simulink model "Wind_Turbine_test"  (R2023b)
settings: Solver=VariableStepAuto  StartTime=0.0  StopTime=1  RelTol=1e-3
model workspace (MAT data in the model file):
  Compensation_Ki = 30
  Compensation_Kp = 3
  DC_Ki = 400
  DC_Kp = 8
  F = 0.01
  Flux_min = 0.5
  Grid_Freq_PWM = 2700
  Grid_Ireg_Ki = 5
  Grid_Ireg_Kp = 0.83
  Grid_Ireg_lim = 1.1
  Grid_Modindex_Upper = 1.1
  Grid_conv_Imax = 0.8
  H = 0.685
  Idref_max = 0.9
  Iqref_Tc = 0.3
  Ki_Var = 0.05
  Ki_Vreg = 20
  Ksh = 1.1
  L_pu = 0.3
  Llr = 0.16
  Lls = 0.18
  Lm = 2.9
  P_mech = 1080000
  Pitch_Ki = 0
  Pitch_Kp = 150
  Pitch_Max = 27
  Pitch_Tc = 0.01
  Pitch_rate = 10
  Q_Filt = 50
  R_pu = 0.003
  Rotor_Freq_PWM = 1620
  Rotor_Ireg_Ki = 8
  Rotor_Ireg_Kp = 0.6
  Rotor_Ireg_lim = 0.1
  Rotor_Modindex_Upper = 2
  Rr = 0.016
  Rs = 0.023
  T_set = 0.0001
  Tp = 5e-05
  Ts = 5e-06
  Var_C_Filt = 720000
  Var_reg_max = 1.1
  Var_reg_min = 0.9
  WT_Coeff = [0.645 116 0.4 5 21 0.00912 0.08 0.035]
  WT_H = 4.32
  WT_IGBTRon = 5.931
  WT_Param = [91.204 10143]
  Wind_Freq_Filt = 10000
  Wind_Freq_nom = 60
  Wind_P_nom = 1200000
  Wind_Rotor_V_nom = 1950
  Wind_V_nom = 500
  Zeta_Filt = 0.707106781187
  init = [-0.2 0 0 0 0 0 0 0]
  p = 3
  torque0 = 0.83
  v_Ki = 0.1
  v_Kp = 3.6
  v_Max = 1.2
  v_Min = 0.7
  v_T = 5
  vreg_max = 1
  wind_VDC_nom = 1150
  wt0 = 1.2
undefined symbols (not defined in the file): D1, D11, Delta, DiscIntNeverNeededParam, P, Q
libraries: powerlib_extras x144, simulink_extras x24, spsThreePhaseVIMeasurementLib x13, spsThreePhaseTransformerTwoWindingsLib x11, spsSeriesRLCBranchLib x9, spsPWMGenerator2LevelLib x8, spsUniversalBridgeLib x8, spsThreePhaseSeriesRLCLoadLib x6, spsThreePhasePISectionLineLib x5, spsGroundLib x5, spsLoadFlowBusLib x4, spsAsynchronousMachinepuUnitsLib x4
(part 1 of 9)
settings Model: Creator=3.22  LastModifiedBy=3.22

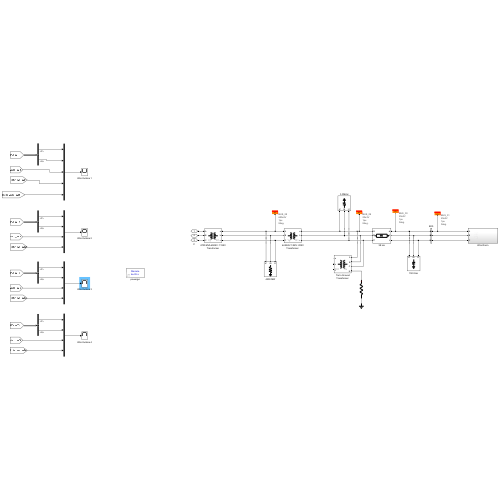
[thumbnail: Simulink's stored preview of the top-level diagram]
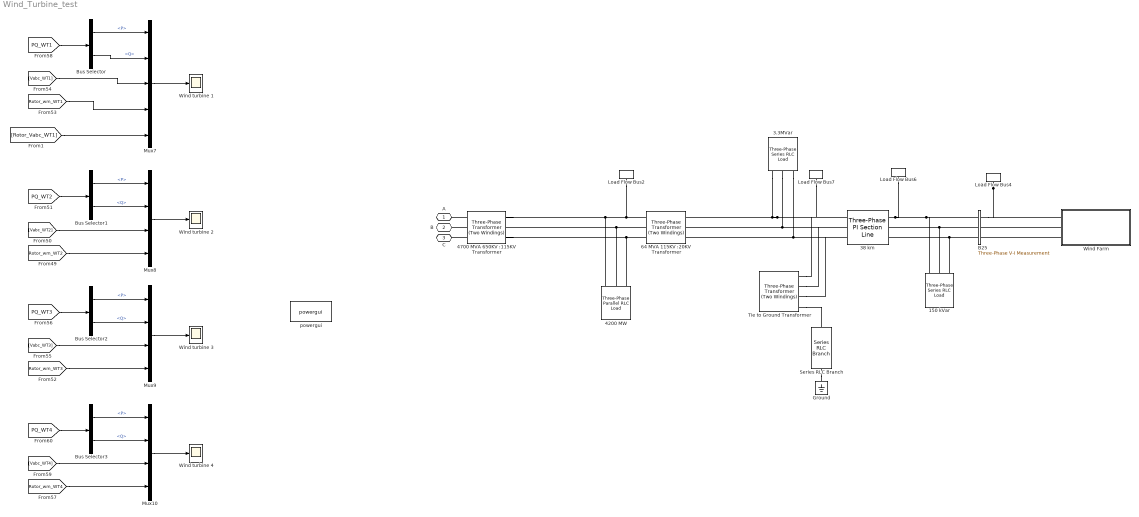
== system Wind_Turbine_test ==
  " 64 MVA 115KV :20KV Transformer " : spsThreePhaseTransformerTwoWindingsLib/Three-Phase Transformer (Two Windings)  Winding1Connection=Yg  Winding2Connection=Delta (D1)  CoreType=Three single-phase transformers  SetSaturation=off  Hysteresis=off  DataFile='hysteresis'  SetInitialFlux=off  Measurements=None  UNITS=pu  NominalPower=[ 64e6 , 60 ]  Winding1=[ 115e3 , 0.002 , 0.08 ]  Winding2=[ 20e3 , 0.002 , 0.08 ]  Rm=500  Lm=500  L0=0.5  Saturation=[ 0,0 ; 0.0024,1.2 ; 1.0,1.52 ]  InitialFluxes=[ 0.8 , -0.8 , 0.7 ]  BreakLoop=off  DiscreteSolver=Trapezoidal iterative  DataType=off  TransfoNumber=1
  " Tie to Ground Transformer " : spsThreePhaseTransformerTwoWindingsLib/Three-Phase Transformer (Two Windings)  Winding1Connection=Yn  Winding2Connection=Delta (D11)  CoreType=Three single-phase transformers  SetSaturation=off  Hysteresis=off  DataFile='hysteresis'  SetInitialFlux=off  Measurements=None  UNITS=pu  NominalPower=[ 5600e6 , 60 ]  Winding1=[ 13.8e3 , 0.002 , 0.08 ]  Winding2=[ 735e3 , 0.002 , 0.08 ]  Rm=500  Lm=500  L0=0.5  Saturation=[ 0,0 ; 0.0024,1.2 ; 1.0,1.52 ]  InitialFluxes=[ 0.8 , -0.8 , 0.7 ]  BreakLoop=off  DiscreteSolver=Trapezoidal iterative  DataType=off  TransfoNumber=1
  150 kVar : spsThreePhaseSeriesRLCLoadLib/Three-Phase Series RLC Load  LConnTagsString=A|B|C  Configuration=Y (grounded)  NominalVoltage=20e3  Vabc=[1e3 1e3 1e3]  Vabcp=[1e3 1e3 1e3]  NominalFrequency=60  UnbalancedPower=off  ActivePower=0  InductivePower=0  CapacitivePower=3.3e6  Pabc=[10e3 9e3 11e3]  QLabc=[100 90 110]  QCabc=[100 90 110]  Pabcp=[10e3 9e3 11e3]  QLabcp=[100 90 110]  QCabcp=[100 90 110]  Measurements=None  LoadType=constant Z
  3.3MVar : spsThreePhaseSeriesRLCLoadLib/Three-Phase Series RLC Load  LConnTagsString=A|B|C  Configuration=Y (grounded)  NominalVoltage=20e3  Vabc=[1e3 1e3 1e3]  Vabcp=[1e3 1e3 1e3]  NominalFrequency=60  UnbalancedPower=off  ActivePower=0  InductivePower=0  CapacitivePower=3.3e6  Pabc=[10e3 9e3 11e3]  QLabc=[100 90 110]  QCabc=[100 90 110]  Pabcp=[10e3 9e3 11e3]  QLabcp=[100 90 110]  QCabcp=[100 90 110]  Measurements=None  LoadType=constant Z
  38 km : spsThreePhasePISectionLineLib/Three-Phase PI Section Line  LConnTagsString=a|b|c  RConnTagsString=A|B|C  Length=38  Frequency=60  Resistances=[ 0.01273 0.3864]/6  Inductances="[ 0.9337e-3  4.1264e-3]/6"  Capacitances=[12.74e-9 7.751e-9]*6
  4200 MW : spsThreePhaseParallelRLCLoadLib/Three-Phase Parallel RLC Load  LConnTagsString=A|B|C  Configuration=Y (grounded)  NominalVoltage=115e3  Vabc=[1e3 1e3 1e3]  Vabcp=[1e3 1e3 1e3]  NominalFrequency=60  UnbalancedPower=off  ActivePower=4.2e6  InductivePower=0  CapacitivePower=0  Pabc=[10e3 9e3 11e3]  QLabc=[100 90 110]  QCabc=[100 90 110]  Pabcp=[10e3 9e3 11e3]  QLabcp=[100 90 110]  QCabcp=[100 90 110]  Measurements=None  LoadType=constant Z
  "4700 MVA 650KV :115KV Transformer " : spsThreePhaseTransformerTwoWindingsLib/Three-Phase Transformer (Two Windings)  Winding1Connection=Yg  Winding2Connection=Delta (D1)  CoreType=Three single-phase transformers  SetSaturation=off  Hysteresis=off  DataFile='hysteresis'  SetInitialFlux=off  Measurements=None  UNITS=pu  NominalPower=[ 4700e6 , 60 ]  Winding1=[ 650e3 , 0.002 , 0.08 ]  Winding2=[ 115e3 , 0.002 , 0.08 ]  Rm=500  Lm=500  L0=0.5  Saturation=[ 0,0 ; 0.0024,1.2 ; 1.0,1.52 ]  InitialFluxes=[ 0.8 , -0.8 , 0.7 ]  BreakLoop=off  DiscreteSolver=Trapezoidal iterative  DataType=off  TransfoNumber=1
  B25 : spsThreePhaseVIMeasurementLib/Three-Phase V-I Measurement  VoltageMeasurement=no  SetLabelV=off  LabelV=Vabc  Vpu=off  VpuLL=off  CurrentMeasurement=no  SetLabelI=off  LabelI=Iabc  Ipu=off  Pbase=100e6  Vbase=500e3  OutputType=Complex  PhasorSimulation=off  PSBequivalent=0
  Bus Selector{,1..3} (4 alike) : BusSelector  OutputSignals=P,Q
  Ground : spsGroundLib/Ground  LConnTagsString=a
  Load Flow Bus2 : spsLoadFlowBusLib/Load Flow Bus  LConnTagsString=a  Phases=single  Connectors=on one side  ID=BUS_28  Vbase=650e3  Vref=1  Vangle=0  VLF=1  VLFb=1  VLFc=1  angleLF=0  angleLFb=0  angleLFc=0
  Load Flow Bus4 : spsLoadFlowBusLib/Load Flow Bus  LConnTagsString=a  Phases=single  Connectors=on one side  ID=BUS_31  Vbase=20e3  Vref=1  Vangle=0  VLF=1  VLFb=1  VLFc=1  angleLF=0  angleLFb=0  angleLFc=0
  Load Flow Bus6 : spsLoadFlowBusLib/Load Flow Bus  LConnTagsString=a  Phases=single  Connectors=on one side  ID=BUS_30  Vbase=20e3  Vref=1  Vangle=0  VLF=1  VLFb=1  VLFc=1  angleLF=0  angleLFb=0  angleLFc=0
  Load Flow Bus7 : spsLoadFlowBusLib/Load Flow Bus  LConnTagsString=a  Phases=single  Connectors=on one side  ID=BUS_29  Vbase=20e3  Vref=1  Vangle=0  VLF=1  VLFb=1  VLFc=1  angleLF=0  angleLFb=0  angleLFc=0
  Mux10 : Mux
  Mux7 : Mux  Inputs=5
  Mux8 : Mux
  Mux9 : Mux
  Series RLC Branch : spsSeriesRLCBranchLib/Series RLC Branch  LConnTagsString=__new0  RConnTagsString=__new0  BranchType=R  Resistance=4.1  Inductance=0  SetiL0=off  InitialCurrent=0  Capacitance=0  Setx0=off  InitialVoltage=0  Measurements=None
  Wind Farm : Subsystem
  Wind turbine {1..4} (4 alike) : Scope
  powergui : sps_lib/powergui  Priority=1  SimulationMode=Discrete  SampleTime=6e-5  frequency=60  Iterations=50  frequencyindice=60  Pbase=100e6  ErrMax=1e-4  UnitsV=kV  UnitsW=MW  buscounter=0  FunctionMessages=off  echomessages=off  EnableUseOfTLC=off  CurrentSourceSwitches=off  DisableSnubberDevices=off  DisableRonSwitches=off  DisableVfSwitches=off  DisplayEquations=off  AutomaticDiscreteSolvers=off  SolverType=Tustin/Backward Euler (TBE)  Interpol=off  ExternalGateDelay=off  methode=off  Ts=100  x0status=blocks  SPID=on  SwTol=0  HookPort=off  NonlinearTolerance=1e-4  nMaxIteration=100  ContinueOnMaxIteration=off  RestoreLinks=warning  ResistiveCurrentMeasurement=off  Frange=[0:2:500]  Ylog=off  Xlog=on  ShowGrid=off  save=off  variable=ZData  structure=0  ZoomFFT=off  StartTime=0.0  cycles=1  DisplayStyle=1  fundamental=60  FreqAxis=off  MaxFrequency=1000  frequencyindicesteady=1  RmsSteady=1  display=off
  A : PMIOPort  Side=Left
  B : PMIOPort  Port=2  Side=Left
  C : PMIOPort  Port=3  Side=Left
  wires:
  [Rotor_wm_WT1] -> Mux7/4
  Bus Selector/1 -> Mux7/1  "<P>"
  [PQ_WT1] -> Bus Selector/1
  Bus Selector/2 -> Mux7/2  "<Q>"
  [Vabc_WT1] -> Mux7/3
  Mux7/1 -> Wind turbine 1/1
  [Rotor_Vabc_WT1] -> Mux7/5
  Mux10/1 -> Wind turbine 4/1
  Bus Selector1/1 -> Mux8/1  "<P>"
  [Rotor_wm_WT2] -> Mux8/4
  Bus Selector3/2 -> Mux10/2  "<Q>"
  Bus Selector1/2 -> Mux8/2  "<Q>"
  [Rotor_wm_WT4] -> Mux10/4
  Mux8/1 -> Wind turbine 2/1
  [Vabc_WT4] -> Mux10/3
  [Vabc_WT3] -> Mux9/3
  Bus Selector3/1 -> Mux10/1  "<P>"
  Bus Selector2/2 -> Mux9/2  "<Q>"
  Mux9/1 -> Wind turbine 3/1
  [Rotor_wm_WT3] -> Mux9/4
  [PQ_WT2] -> Bus Selector1/1
  [PQ_WT3] -> Bus Selector2/1
  [PQ_WT4] -> Bus Selector3/1
  Bus Selector2/1 -> Mux9/1  "<P>"
  [Vabc_WT2] -> Mux8/3
  connections:
  4200 MW/LConn3 -- "4700 MVA 650KV :115KV Transformer "/RConn3 -- " 64 MVA 115KV :20KV Transformer "/LConn3
  38 km/RConn1 -- Load Flow Bus6/LConn1 -- 150 kVar/LConn1 -- B25/RConn1
  Load Flow Bus4/LConn1 -- Wind Farm/LConn1 -- B25/LConn1
  3.3MVar/LConn1 -- 38 km/LConn1 -- Load Flow Bus7/LConn1 -- " Tie to Ground Transformer "/LConn1 -- " 64 MVA 115KV :20KV Transformer "/RConn1
  3.3MVar/LConn2 -- 38 km/LConn2 -- " Tie to Ground Transformer "/LConn2 -- " 64 MVA 115KV :20KV Transformer "/RConn2
  3.3MVar/LConn3 -- " 64 MVA 115KV :20KV Transformer "/RConn3 -- 38 km/LConn3 -- " Tie to Ground Transformer "/LConn3
  B25/RConn3 -- 150 kVar/LConn3 -- 38 km/RConn3
  4200 MW/LConn2 -- "4700 MVA 650KV :115KV Transformer "/RConn2 -- " 64 MVA 115KV :20KV Transformer "/LConn2
  Load Flow Bus2/LConn1 -- "4700 MVA 650KV :115KV Transformer "/RConn1 -- 4200 MW/LConn1 -- " 64 MVA 115KV :20KV Transformer "/LConn1
  B25/RConn2 -- 150 kVar/LConn2 -- 38 km/RConn2
  Series RLC Branch/RConn1 -- Ground/LConn1
  Wind Farm/LConn3 -- B25/LConn3
  Wind Farm/LConn2 -- B25/LConn2
  " Tie to Ground Transformer "/LConn4 -- Series RLC Branch/LConn1
  "4700 MVA 650KV :115KV Transformer "/LConn3 -- C/RConn1
  "4700 MVA 650KV :115KV Transformer "/LConn1 -- A/RConn1
  "4700 MVA 650KV :115KV Transformer "/LConn2 -- B/RConn1

== system Wind_Turbine_test/Wind Farm ==
  12 MVA 20KV :575V Transformer {1..4} (4 alike) : spsThreePhaseTransformerTwoWindingsLib/Three-Phase Transformer (Two Windings)  Winding1Connection=Delta (D1)  Winding2Connection=Yn  CoreType=Three single-phase transformers  SetSaturation=off  Hysteresis=off  DataFile='hysteresis'  SetInitialFlux=off  Measurements=None  UNITS=pu  NominalPower=[ 1.15e7 , 60 ]  Winding1=[ 20e3 , 0.002 , 0.08 ]  Winding2=[ 500 , 0.002 , 0.08 ]  Rm=500  Lm=500  L0=0.5  Saturation=[ 0,0 ; 0.0024,1.2 ; 1.0,1.52 ]  InitialFluxes=[ 0.8 , -0.8 , 0.7 ]  BreakLoop=off  DiscreteSolver=Trapezoidal iterative  DataType=off  TransfoNumber=1
  Control System : Subsystem
  Ground{,1..3} (4 alike) : spsGroundLib/Ground  LConnTagsString=a
  Series RLC Branch{,1..3} (4 alike) : spsSeriesRLCBranchLib/Series RLC Branch  LConnTagsString=__new0  RConnTagsString=__new0  BranchType=R  Resistance=66  Inductance=0  SetiL0=off  InitialCurrent=0  Capacitance=0  Setx0=off  InitialVoltage=0  Measurements=None
  Three-Phase PI Section Line{,1..3} (4 alike) : spsThreePhasePISectionLineLib/Three-Phase PI Section Line  LConnTagsString=a|b|c  RConnTagsString=A|B|C  Length=0.5  Frequency=60  Resistances=[ 0.01273 0.3864]  Inductances="[ 0.9337e-3  4.1264e-3]"  Capacitances=[12.74e-9 7.751e-9]
  Three-Phase Series RLC Load{,1..3} (4 alike) : spsThreePhaseSeriesRLCLoadLib/Three-Phase Series RLC Load  LConnTagsString=A|B|C  Configuration=Y (grounded)  NominalVoltage=500  Vabc=[1e3 1e3 1e3]  Vabcp=[1e3 1e3 1e3]  NominalFrequency=60  UnbalancedPower=off  ActivePower=43200  InductivePower=0  CapacitivePower=2160e3  Pabc=[10e3 9e3 11e3]  QLabc=[100 90 110]  QCabc=[100 90 110]  Pabcp=[10e3 9e3 11e3]  QLabcp=[100 90 110]  QCabcp=[100 90 110]  Measurements=None  LoadType=constant Z
  Three-Phase V-I Measurement1 : spsThreePhaseVIMeasurementLib/Three-Phase V-I Measurement  VoltageMeasurement=phase-to-ground  SetLabelV=on  LabelV=Vabc_WT2  Vpu=on  VpuLL=off  CurrentMeasurement=no  SetLabelI=on  LabelI=Iabc_WT2  Ipu=on  Pbase=2*1.8/0.9  Vbase=500  OutputType=Complex  PhasorSimulation=off  PSBequivalent=0
  Three-Phase V-I Measurement2 : spsThreePhaseVIMeasurementLib/Three-Phase V-I Measurement  VoltageMeasurement=phase-to-ground  SetLabelV=on  LabelV=Vabc_WT1  Vpu=on  VpuLL=off  CurrentMeasurement=no  SetLabelI=on  LabelI=Iabc_WT1  Ipu=off  Pbase=2*1.8/0.9  Vbase=500  OutputType=Complex  PhasorSimulation=off  PSBequivalent=0
  Three-Phase V-I Measurement3 : spsThreePhaseVIMeasurementLib/Three-Phase V-I Measurement  VoltageMeasurement=phase-to-ground  SetLabelV=on  LabelV=Vabc_WT4  Vpu=on  VpuLL=off  CurrentMeasurement=no  SetLabelI=on  LabelI=Iabc_WT4  Ipu=on  Pbase=2*1.8/0.9  Vbase=500  OutputType=Complex  PhasorSimulation=off  PSBequivalent=0
  Three-Phase V-I Measurement4 : spsThreePhaseVIMeasurementLib/Three-Phase V-I Measurement  VoltageMeasurement=phase-to-ground  SetLabelV=on  LabelV=Vabc_WT3  Vpu=on  VpuLL=off  CurrentMeasurement=no  SetLabelI=on  LabelI=Iabc_WT3  Ipu=on  Pbase=2*1.8/0.9  Vbase=500  OutputType=Complex  PhasorSimulation=off  PSBequivalent=0
  Unit Delay1 : UnitDelay  SampleTime=Ts  HasFrameUpgradeWarning=on
  Wind Turbine 1 : Subsystem
  Wind Turbine 2 : Subsystem
  Wind Turbine 3 : Subsystem
  Wind Turbine 4 : Subsystem
  A : PMIOPort  Side=Left
  B : PMIOPort  Port=2  Side=Left
  C : PMIOPort  Port=3  Side=Left
  connections:
  Three-Phase PI Section Line/RConn1 -- 12 MVA 20KV :575V Transformer 1/LConn1
  12 MVA 20KV :575V Transformer 1/LConn2 -- Three-Phase PI Section Line/RConn2
  Three-Phase PI Section Line/RConn3 -- 12 MVA 20KV :575V Transformer 1/LConn3
  Ground/LConn1 -- Series RLC Branch/RConn1
  Series RLC Branch/LConn1 -- 12 MVA 20KV :575V Transformer 1/RConn4
  12 MVA 20KV :575V Transformer 2/RConn1 -- Three-Phase V-I Measurement1/LConn1
  12 MVA 20KV :575V Transformer 2/RConn3 -- Three-Phase V-I Measurement1/LConn3
  12 MVA 20KV :575V Transformer 2/RConn2 -- Three-Phase V-I Measurement1/LConn2
  12 MVA 20KV :575V Transformer 2/RConn4 -- Series RLC Branch1/LConn1
  12 MVA 20KV :575V Transformer 2/LConn2 -- Three-Phase PI Section Line1/RConn2
  12 MVA 20KV :575V Transformer 2/LConn1 -- Three-Phase PI Section Line1/RConn1
  12 MVA 20KV :575V Transformer 2/LConn3 -- Three-Phase PI Section Line1/RConn3
  Ground1/LConn1 -- Series RLC Branch1/RConn1
  12 MVA 20KV :575V Transformer 3/RConn1 -- Three-Phase V-I Measurement4/LConn1
  12 MVA 20KV :575V Transformer 3/RConn3 -- Three-Phase V-I Measurement4/LConn3
  12 MVA 20KV :575V Transformer 3/RConn2 -- Three-Phase V-I Measurement4/LConn2
  12 MVA 20KV :575V Transformer 3/RConn4 -- Series RLC Branch2/LConn1
  12 MVA 20KV :575V Transformer 3/LConn2 -- Three-Phase PI Section Line2/RConn2
  12 MVA 20KV :575V Transformer 3/LConn1 -- Three-Phase PI Section Line2/RConn1
  12 MVA 20KV :575V Transformer 3/LConn3 -- Three-Phase PI Section Line2/RConn3
  Ground2/LConn1 -- Series RLC Branch2/RConn1
  12 MVA 20KV :575V Transformer 4/RConn1 -- Three-Phase V-I Measurement3/LConn1
  12 MVA 20KV :575V Transformer 4/RConn3 -- Three-Phase V-I Measurement3/LConn3
  12 MVA 20KV :575V Transformer 4/RConn2 -- Three-Phase V-I Measurement3/LConn2
  12 MVA 20KV :575V Transformer 4/RConn4 -- Series RLC Branch3/LConn1
  12 MVA 20KV :575V Transformer 4/LConn2 -- Three-Phase PI Section Line3/RConn2
  12 MVA 20KV :575V Transformer 4/LConn1 -- Three-Phase PI Section Line3/RConn1
  12 MVA 20KV :575V Transformer 4/LConn3 -- Three-Phase PI Section Line3/RConn3
  Ground3/LConn1 -- Series RLC Branch3/RConn1
  Three-Phase PI Section Line3/LConn1 -- Three-Phase PI Section Line/LConn1 -- Three-Phase PI Section Line1/LConn1 -- A/RConn1 -- Three-Phase PI Section Line2/LConn1
  Three-Phase PI Section Line3/LConn2 -- Three-Phase PI Section Line2/LConn2 -- Three-Phase PI Section Line/LConn2 -- Three-Phase PI Section Line1/LConn2 -- B/RConn1
  Three-Phase PI Section Line3/LConn3 -- Three-Phase PI Section Line2/LConn3 -- Three-Phase PI Section Line/LConn3 -- Three-Phase PI Section Line1/LConn3 -- C/RConn1
  Wind Turbine 2/LConn3 -- Three-Phase Series RLC Load1/LConn3 -- Three-Phase V-I Measurement1/RConn3
  Wind Turbine 2/LConn2 -- Three-Phase Series RLC Load1/LConn2 -- Three-Phase V-I Measurement1/RConn2
  Three-Phase V-I Measurement1/RConn1 -- Three-Phase Series RLC Load1/LConn1 -- Wind Turbine 2/LConn1
  Wind Turbine 3/LConn3 -- Three-Phase Series RLC Load2/LConn3 -- Three-Phase V-I Measurement4/RConn3
  Wind Turbine 3/LConn2 -- Three-Phase Series RLC Load2/LConn2 -- Three-Phase V-I Measurement4/RConn2
  Wind Turbine 3/LConn1 -- Three-Phase Series RLC Load2/LConn1 -- Three-Phase V-I Measurement4/RConn1
  Wind Turbine 4/LConn3 -- Three-Phase Series RLC Load3/LConn3 -- Three-Phase V-I Measurement3/RConn3
  Wind Turbine 4/LConn2 -- Three-Phase Series RLC Load3/LConn2 -- Three-Phase V-I Measurement3/RConn2
  Three-Phase V-I Measurement3/RConn1 -- Three-Phase Series RLC Load3/LConn1 -- Wind Turbine 4/LConn1
  Three-Phase V-I Measurement2/LConn1 -- 12 MVA 20KV :575V Transformer 1/RConn1
  Three-Phase V-I Measurement2/LConn2 -- 12 MVA 20KV :575V Transformer 1/RConn2
  Three-Phase V-I Measurement2/LConn3 -- 12 MVA 20KV :575V Transformer 1/RConn3
  Three-Phase V-I Measurement2/RConn1 -- Wind Turbine 1/LConn1 -- Three-Phase Series RLC Load/LConn1
  Three-Phase V-I Measurement2/RConn2 -- Wind Turbine 1/LConn2 -- Three-Phase Series RLC Load/LConn2
  Three-Phase V-I Measurement2/RConn3 -- Wind Turbine 1/LConn3 -- Three-Phase Series RLC Load/LConn3

== system Wind_Turbine_test/Wind Farm/Control System ==
  Control System 1 : Subsystem
  Control System 2 : Subsystem
  Control System 3 : Subsystem
  Control System 4 : Subsystem
  tag scope: Grid_conv_pulses_WT1=global, Grid_conv_pulses_WT2=global, Grid_conv_pulses_WT3=global, Grid_conv_pulses_WT4=global, PQ_WT1=global, PQ_WT2=global, PQ_WT3=global, PQ_WT4=global, Pitch_WT1=global, Pitch_WT2=global, Pitch_WT3=global, Pitch_WT4=global, Rotor_conv_pulses_WT1=global, Rotor_conv_pulses_WT2=global, Rotor_conv_pulses_WT3=global, Rotor_conv_pulses_WT4=global
  wires:
  [Vabc_WT1] -> Control System 1/1(Vabc)
  Control System 4/1(Grid_conv_pulses) -> [Grid_conv_pulses_WT4]
  [Stator_Iabc_WT4] -> Control System 4/2(Stator_Iabc)
  [Grid_conv_Iabc_WT3] -> Control System 3/3(Grid_Iabc)
  [Q_ref_WT2] -> Control System 2/6(Qref1)
  [Rotor_wm_WT1] -> Control System 1/8(wr)
  Control System 1/3(Pitch) -> [Pitch_WT1]
  Control System 2/1(Grid_conv_pulses) -> [Grid_conv_pulses_WT2]
  Control System 2/2(Rotor_conv_pulses) -> [Rotor_conv_pulses_WT2]
  [Rotor_Iabc_WT3] -> Control System 3/4(Rotor_Iabc)
  [Grid_conv_Iabc_WT1] -> Control System 1/3(Grid_Iabc)
  Control System 4/3(Pitch) -> [Pitch_WT4]
  Control System 4/2(Rotor_conv_pulses) -> [Rotor_conv_pulses_WT4]
  [VDC_WT2] -> Control System 2/5(Vdc_V)
  [Rotor_Angle_WT1] -> Control System 1/7(angle_rotor_rad)
  [Q_ref_WT1] -> Control System 1/6(Qref1)
  [VDC_WT3] -> Control System 3/5(Vdc_V)
  Control System 3/3(Pitch) -> [Pitch_WT3]
  [Stator_Iabc_WT3] -> Control System 3/2(Stator_Iabc)
  [Rotor_wm_WT3] -> Control System 3/8(wr)
  [Rotor_Angle_WT3] -> Control System 3/7(angle_rotor_rad)
  [Stator_Iabc_WT1] -> Control System 1/2(Stator_Iabc)
  [Q_ref_WT3] -> Control System 3/6(Qref1)
  [Vabc_WT2] -> Control System 2/1(Vabc)
  [Vabc_WT3] -> Control System 3/1(Vabc)
  [Rotor_Iabc_WT1] -> Control System 1/4(Rotor_Iabc)
  [Rotor_Angle_WT2] -> Control System 2/7(angle_rotor_rad)
  [Stator_Iabc_WT2] -> Control System 2/2(Stator_Iabc)
  [Grid_conv_Iabc_WT2] -> Control System 2/3(Grid_Iabc)
  [VDC_WT4] -> Control System 4/5(Vdc_V)
  [Rotor_Iabc_WT2] -> Control System 2/4(Rotor_Iabc)
  [Vabc_WT4] -> Control System 4/1(Vabc)
  [Grid_conv_Iabc_WT4] -> Control System 4/3(Grid_Iabc)
  [Rotor_wm_WT2] -> Control System 2/8(wr)
  [Rotor_Iabc_WT4] -> Control System 4/4(Rotor_Iabc)
  Control System 1/2(Rotor_conv_pulses) -> [Rotor_conv_pulses_WT1]
  Control System 2/3(Pitch) -> [Pitch_WT2]
  [VDC_WT1] -> Control System 1/5(Vdc_V)
  Control System 3/1(Grid_conv_pulses) -> [Grid_conv_pulses_WT3]
  Control System 1/1(Grid_conv_pulses) -> [Grid_conv_pulses_WT1]
  Control System 3/2(Rotor_conv_pulses) -> [Rotor_conv_pulses_WT3]
  [Q_ref_WT4] -> Control System 4/6(Qref1)
  [Rotor_Angle_WT4] -> Control System 4/7(angle_rotor_rad)
  [Rotor_wm_WT4] -> Control System 4/8(wr)
  Control System 1/4(PQ) -> [PQ_WT1]
  Control System 2/4(PQ) -> [PQ_WT2]
  Control System 3/4(PQ) -> [PQ_WT3]
  Control System 4/4(PQ) -> [PQ_WT4]

== system Wind_Turbine_test/Wind Farm/Wind Turbine 1 ==
  " base " : Gain  Gain=-P_mech/Wind_P_nom  SaturateOnIntegerOverflow=on  OutDataTypeStr=Inherit: Same as input  ParamDataTypeStr=Inherit: Same as input
  Asynchronous Machine pu Units : spsAsynchronousMachinepuUnitsLib/Asynchronous Machine pu Units  RotorType=Wound  PresetModel=No  MechanicalLoad=Torque Tm  ShowDetailedParameters=on  ReferenceFrame=Rotor  Units=pu  MeasurementBus=off  NominalParameters=[1.15e7 500 60]  VoltageRatio=1  Stator=[0.023 0.18]  Rotor=[0.016 0.16]  Cage1=[0.01909 0.0397]  Cage2=[0.01909 0.0397]  Lm=2.9  Mechanical=[0.685,0.01,3]  PolePairs=2  InitialConditions="[ -0.2,0   0,0,0   0,0,0 ]"  SimulateSaturation=off  Saturation="[0.212,0.4201,0.8125,1.0979,1.4799,2.2457,3.2586,4.5763,6.4763 ;   0.5,0.7,0.9,1,1.1,1.2 ,1.3,1.4,1.5]"  LoadFlowParameters=0  TsPowergui=0  TsBlock=-1  IterativeModel=Trapezoidal non iterative  IterativeDiscreteModel=Trapezoidal non iterative  Pmec=1.08e6
      settings: LibrarySourceBlock=|
      | sps_lib/Electrical Machines/Asynchronous Machine
      | pu Units
  Bus Selector : BusSelector  OutputSignals=Stator measurements.Stator current is_a (pu),Stator measurements.Stator current is_b (pu),Stator measurements.Stator current is_c (pu),Rotor measurements.Rotor current ir_a (pu),Rotor measurements.Rotor current ir_b (pu),Rotor measurements.Rotor current ir_c (pu),Mechanical.Electromagnetic torque Te (pu),Mechanical.Rotor speed (wm),Mechanical.Rotor angle thetam (rad)
  Mux : Mux  Inputs=3
  Mux1 : Mux  Inputs=3
  Scope : Scope
  Series RLC Branch4 : spsSeriesRLCBranchLib/Series RLC Branch  LConnTagsString=__new0  RConnTagsString=__new0  BranchType=C  Resistance=1  Inductance=1e-3  SetiL0=off  InitialCurrent=0  Capacitance=0.06  Setx0=on  InitialVoltage=1175  Measurements=None
  Three-Phase Series RLC Branch : spsThreePhaseSeriesRLCBranchLib/Three-Phase Series RLC Branch  LConnTagsString=A|B|C  RConnTagsString=A|B|C  BranchType=RL  Resistance=(Wind_V_nom^2/Wind_P_nom)*R_pu  Inductance=(Wind_V_nom^2/Wind_P_nom/(2*pi*Wind_Freq_nom))*L_pu  Capacitance=1e-6  Measurements=None
  Three-Phase Transformer (Two Windings) : spsThreePhaseTransformerTwoWindingsLib/Three-Phase Transformer (Two Windings)  Winding1Connection=Y  Winding2Connection=Y  CoreType=Three single-phase transformers  SetSaturation=off  Hysteresis=off  DataFile='hysteresis'  SetInitialFlux=off  Measurements=None  UNITS=pu  NominalPower=[1.15e7, 60 ]  Winding1="[ 500, 0,0  ]"  Winding2=[ 1950 , 0 , 0 ]  Rm=500  Lm=inf  L0=0.5  Saturation=[ 0,0 ; 0.0024,1.2 ; 1.0,1.52 ]  InitialFluxes=[ 0.8 , -0.8 , 0.7 ]  BreakLoop=off  DiscreteSolver=Trapezoidal iterative  DataType=off  TransfoNumber=1
  Three-Phase V-I Measurement5 : spsThreePhaseVIMeasurementLib/Three-Phase V-I Measurement  VoltageMeasurement=phase-to-ground  SetLabelV=on  LabelV=Rotor_Vabc_WT1  Vpu=on  VpuLL=off  CurrentMeasurement=no  SetLabelI=on  LabelI=Iabc_WT1  Ipu=on  Pbase=2*1.8/0.9  Vbase=Wind_Rotor_V_nom  OutputType=Complex  PhasorSimulation=off  PSBequivalent=0
  Three-Phase V-I Measurement6 : spsThreePhaseVIMeasurementLib/Three-Phase V-I Measurement  VoltageMeasurement=phase-to-ground  SetLabelV=on  LabelV=Grid_conv_Vabc_WT1  Vpu=on  VpuLL=off  CurrentMeasurement=yes  SetLabelI=on  LabelI=Grid_conv_Iabc_WT1  Ipu=on  Pbase=1.15e7  Vbase=Wind_V_nom  OutputType=Complex  PhasorSimulation=off  PSBequivalent=0
  Universal Bridge : spsUniversalBridgeLib/Universal Bridge  Arms=3  SnubberResistance=1e3  SnubberCapacitance=inf  Device=IGBT / Diodes  Ron=1e-4/WT_IGBTRon  Lon=0  ForwardVoltages="[  0  0  ]"  ForwardVoltage=0  GTOparameters=[ 10e-6 , 20e-6 ]  IGBTparameters=[ 1e-6 , 2e-6 ]  Measurements=None  Measurements_2=None  converterType=Rectifier
  Universal Bridge1 : spsUniversalBridgeLib/Universal Bridge  Arms=3  SnubberResistance=1e3  SnubberCapacitance=inf  Device=IGBT / Diodes  Ron=1e-4/WT_IGBTRon  Lon=0  ForwardVoltages="[  0  0  ]"  ForwardVoltage=0  GTOparameters=[ 10e-6 , 20e-6 ]  IGBTparameters=[ 1e-6 , 2e-6 ]  Measurements=None  Measurements_2=None  converterType=Rectifier
  Wind Turbine & Generator 1 : Subsystem
  A : PMIOPort  Side=Left
  B : PMIOPort  Port=2  Side=Left
  C : PMIOPort  Port=3  Side=Left
  tag scope: Rotor_Angle_WT1=global, Rotor_Iabc_WT1=global, Rotor_Tem_WT1=global, Rotor_wm_WT1=global, Stator_Iabc_WT1=global, Tshaft_WT1=global, m_WT1=global
  wires:
  [Tshaft_WT1] -> Asynchronous Machine pu Units/1
  Wind Turbine & Generator 1/1(T_shaft (pu)) -> " base "/1
  " base "/1 -> Scope/1, [Tshaft_WT1]
  Asynchronous Machine pu Units/1 -> [m_WT1]
  [Grid_conv_pulses_WT1] -> Universal Bridge1/1
  [Rotor_conv_pulses_WT1] -> Universal Bridge/1
  [Rotor_wm_WT1] -> Wind Turbine & Generator 1/1(Generator speed (pu))
  [m_WT1] -> Bus Selector/1
  Bus Selector/1 -> Mux1/1  "<Stator current is_a (pu)>"
  Bus Selector/2 -> Mux1/2  "<Stator current is_b (pu)>"
  Bus Selector/3 -> Mux1/3  "<Stator current is_c (pu)>"
  Bus Selector/4 -> Mux/1  "<Rotor current ir_a (pu)>"
  Bus Selector/5 -> Mux/2  "<Rotor current ir_b (pu)>"
  Bus Selector/6 -> Mux/3  "<Rotor current ir_c (pu)>"
  Bus Selector/7 -> [Rotor_Tem_WT1]  "<Electromagnetic torque Te (pu)>"
  Bus Selector/8 -> [Rotor_wm_WT1]  "<Rotor speed (wm)>"
  Bus Selector/9 -> [Rotor_Angle_WT1]  "<Rotor angle thetam (rad)>"
  Mux/1 -> [Rotor_Iabc_WT1]
  Mux1/1 -> [Stator_Iabc_WT1]
  connections:
  Asynchronous Machine pu Units/LConn3 -- C/RConn1 -- Three-Phase Series RLC Branch/LConn3
  Three-Phase Series RLC Branch/LConn1 -- A/RConn1 -- Asynchronous Machine pu Units/LConn1
  Three-Phase Transformer (Two Windings)/LConn1 -- Asynchronous Machine pu Units/RConn1
  Three-Phase Transformer (Two Windings)/RConn1 -- Three-Phase V-I Measurement5/LConn1
  Three-Phase Series RLC Branch/LConn2 -- B/RConn1 -- Asynchronous Machine pu Units/LConn2
  Universal Bridge1/LConn3 -- Three-Phase V-I Measurement6/RConn3
  Three-Phase Transformer (Two Windings)/LConn3 -- Asynchronous Machine pu Units/RConn3
  Three-Phase Transformer (Two Windings)/LConn2 -- Asynchronous Machine pu Units/RConn2
  Universal Bridge1/LConn2 -- Three-Phase V-I Measurement6/RConn2
  Universal Bridge/RConn1 -- Series RLC Branch4/LConn1 -- Universal Bridge1/RConn1
  Universal Bridge1/RConn2 -- Series RLC Branch4/RConn1 -- Universal Bridge/RConn2
  Three-Phase Transformer (Two Windings)/RConn2 -- Three-Phase V-I Measurement5/LConn2
  Three-Phase V-I Measurement5/RConn3 -- Universal Bridge/LConn3
  Three-Phase V-I Measurement5/RConn1 -- Universal Bridge/LConn1
  Three-Phase Transformer (Two Windings)/RConn3 -- Three-Phase V-I Measurement5/LConn3
  Three-Phase V-I Measurement6/LConn1 -- Three-Phase Series RLC Branch/RConn1
  Three-Phase Series RLC Branch/RConn2 -- Three-Phase V-I Measurement6/LConn2
  Universal Bridge1/LConn1 -- Three-Phase V-I Measurement6/RConn1
  Three-Phase Series RLC Branch/RConn3 -- Three-Phase V-I Measurement6/LConn3
  Three-Phase V-I Measurement5/RConn2 -- Universal Bridge/LConn2

== system Wind_Turbine_test/Wind Farm/Wind Turbine 2 ==
  " base " : Gain  Gain=-P_mech/Wind_P_nom  SaturateOnIntegerOverflow=on  OutDataTypeStr=Inherit: Same as input  ParamDataTypeStr=Inherit: Same as input
  Asynchronous Machine pu Units : spsAsynchronousMachinepuUnitsLib/Asynchronous Machine pu Units  RotorType=Wound  PresetModel=No  MechanicalLoad=Torque Tm  ShowDetailedParameters=on  ReferenceFrame=Rotor  Units=pu  MeasurementBus=off  NominalParameters=[1.15e7 500 60]  VoltageRatio=1  Stator=[0.023 0.18]  Rotor=[0.016 0.16]  Cage1=[0.01909 0.0397]  Cage2=[0.01909 0.0397]  Lm=2.9  Mechanical=[0.685,0.01,3]  PolePairs=2  InitialConditions="[ -0.2,0   0,0,0   0,0,0 ]"  SimulateSaturation=off  Saturation="[0.212,0.4201,0.8125,1.0979,1.4799,2.2457,3.2586,4.5763,6.4763 ;   0.5,0.7,0.9,1,1.1,1.2 ,1.3,1.4,1.5]"  LoadFlowParameters=0  TsPowergui=0  TsBlock=-1  IterativeModel=Trapezoidal non iterative  IterativeDiscreteModel=Trapezoidal non iterative  Pmec=1.08e6
      settings: LibrarySourceBlock=|
      | sps_lib/Electrical Machines/Asynchronous Machine
      | pu Units
  Bus Selector : BusSelector  OutputSignals=Stator measurements.Stator current is_a (pu),Stator measurements.Stator current is_b (pu),Stator measurements.Stator current is_c (pu),Rotor measurements.Rotor current ir_a (pu),Rotor measurements.Rotor current ir_b (pu),Rotor measurements.Rotor current ir_c (pu),Mechanical.Electromagnetic torque Te (pu),Mechanical.Rotor speed (wm),Mechanical.Rotor angle thetam (rad)
  Mux : Mux  Inputs=3
  Mux1 : Mux  Inputs=3
  Series RLC Branch4 : spsSeriesRLCBranchLib/Series RLC Branch  LConnTagsString=__new0  RConnTagsString=__new0  BranchType=C  Resistance=1  Inductance=1e-3  SetiL0=off  InitialCurrent=0  Capacitance=0.06  Setx0=on  InitialVoltage=1175  Measurements=None
  Three-Phase Series RLC Branch : spsThreePhaseSeriesRLCBranchLib/Three-Phase Series RLC Branch  LConnTagsString=A|B|C  RConnTagsString=A|B|C  BranchType=RL  Resistance=(Wind_V_nom^2/Wind_P_nom)*R_pu  Inductance=(Wind_V_nom^2/Wind_P_nom/(2*pi*Wind_Freq_nom))*L_pu  Capacitance=1e-6  Measurements=None
  Three-Phase Transformer (Two Windings) : spsThreePhaseTransformerTwoWindingsLib/Three-Phase Transformer (Two Windings)  Winding1Connection=Y  Winding2Connection=Y  CoreType=Three single-phase transformers  SetSaturation=off  Hysteresis=off  DataFile='hysteresis'  SetInitialFlux=off  Measurements=None  UNITS=pu  NominalPower=[1.15e7, 60 ]  Winding1="[ 500, 0,0  ]"  Winding2=[ 1950 , 0 , 0 ]  Rm=500  Lm=inf  L0=0.5  Saturation=[ 0,0 ; 0.0024,1.2 ; 1.0,1.52 ]  InitialFluxes=[ 0.8 , -0.8 , 0.7 ]  BreakLoop=off  DiscreteSolver=Trapezoidal iterative  DataType=off  TransfoNumber=1
  Three-Phase V-I Measurement5 : spsThreePhaseVIMeasurementLib/Three-Phase V-I Measurement  VoltageMeasurement=phase-to-ground  SetLabelV=on  LabelV=Rotor_Vabc_WT2  Vpu=on  VpuLL=off  CurrentMeasurement=no  SetLabelI=on  LabelI=Iabc_WT1  Ipu=on  Pbase=2*1.8/0.9  Vbase=Wind_Rotor_V_nom  OutputType=Complex  PhasorSimulation=off  PSBequivalent=0
  Three-Phase V-I Measurement6 : spsThreePhaseVIMeasurementLib/Three-Phase V-I Measurement  VoltageMeasurement=phase-to-ground  SetLabelV=on  LabelV=Grid_conv_Vabc_WT2  Vpu=on  VpuLL=off  CurrentMeasurement=yes  SetLabelI=on  LabelI=Grid_conv_Iabc_WT2  Ipu=on  Pbase=1.15e7  Vbase=Wind_V_nom  OutputType=Complex  PhasorSimulation=off  PSBequivalent=0
  Universal Bridge : spsUniversalBridgeLib/Universal Bridge  Arms=3  SnubberResistance=1e3  SnubberCapacitance=inf  Device=IGBT / Diodes  Ron=1e-4/WT_IGBTRon  Lon=0  ForwardVoltages="[  0  0  ]"  ForwardVoltage=0  GTOparameters=[ 10e-6 , 20e-6 ]  IGBTparameters=[ 1e-6 , 2e-6 ]  Measurements=None  Measurements_2=None  converterType=Rectifier
  Universal Bridge1 : spsUniversalBridgeLib/Universal Bridge  Arms=3  SnubberResistance=1e3  SnubberCapacitance=inf  Device=IGBT / Diodes  Ron=1e-4/WT_IGBTRon  Lon=0  ForwardVoltages="[  0  0  ]"  ForwardVoltage=0  GTOparameters=[ 10e-6 , 20e-6 ]  IGBTparameters=[ 1e-6 , 2e-6 ]  Measurements=None  Measurements_2=None  converterType=Rectifier
  Wind Turbine & Generator 1 : Subsystem
  A : PMIOPort  Side=Left
  B : PMIOPort  Port=2  Side=Left
  C : PMIOPort  Port=3  Side=Left
  tag scope: Rotor_Angle_WT2=global, Rotor_Iabc_WT2=global, Rotor_Tem_WT2=global, Rotor_wm_WT2=global, Stator_Iabc_WT2=global, Tshaft_WT2=global, m_WT2=global
  wires:
  [Tshaft_WT2] -> Asynchronous Machine pu Units/1
  Wind Turbine & Generator 1/1(T_shaft (pu)) -> " base "/1
  " base "/1 -> [Tshaft_WT2]
  Asynchronous Machine pu Units/1 -> [m_WT2]
  [Grid_conv_pulses_WT2] -> Universal Bridge1/1
  [Rotor_conv_pulses_WT2] -> Universal Bridge/1
  [Rotor_wm_WT2] -> Wind Turbine & Generator 1/1(Generator speed (pu))
  [m_WT2] -> Bus Selector/1
  Bus Selector/1 -> Mux1/1  "<Stator current is_a (pu)>"
  Bus Selector/2 -> Mux1/2  "<Stator current is_b (pu)>"
  Bus Selector/3 -> Mux1/3  "<Stator current is_c (pu)>"
  Bus Selector/4 -> Mux/1  "<Rotor current ir_a (pu)>"
  Bus Selector/5 -> Mux/2  "<Rotor current ir_b (pu)>"
  Bus Selector/6 -> Mux/3  "<Rotor current ir_c (pu)>"
  Bus Selector/7 -> [Rotor_Tem_WT2]  "<Electromagnetic torque Te (pu)>"
  Bus Selector/8 -> [Rotor_wm_WT2]  "<Rotor speed (wm)>"
  Bus Selector/9 -> [Rotor_Angle_WT2]  "<Rotor angle thetam (rad)>"
  Mux/1 -> [Rotor_Iabc_WT2]
  Mux1/1 -> [Stator_Iabc_WT2]
  connections:
  Asynchronous Machine pu Units/LConn3 -- C/RConn1 -- Three-Phase Series RLC Branch/LConn3
  Three-Phase Series RLC Branch/LConn1 -- A/RConn1 -- Asynchronous Machine pu Units/LConn1
  Three-Phase Transformer (Two Windings)/LConn1 -- Asynchronous Machine pu Units/RConn1
  Three-Phase Transformer (Two Windings)/RConn1 -- Three-Phase V-I Measurement5/LConn1
  Three-Phase Series RLC Branch/LConn2 -- B/RConn1 -- Asynchronous Machine pu Units/LConn2
  Universal Bridge1/LConn3 -- Three-Phase V-I Measurement6/RConn3
  Three-Phase Transformer (Two Windings)/LConn3 -- Asynchronous Machine pu Units/RConn3
  Three-Phase Transformer (Two Windings)/LConn2 -- Asynchronous Machine pu Units/RConn2
  Universal Bridge1/LConn2 -- Three-Phase V-I Measurement6/RConn2
  Universal Bridge/RConn1 -- Series RLC Branch4/LConn1 -- Universal Bridge1/RConn1
  Universal Bridge1/RConn2 -- Series RLC Branch4/RConn1 -- Universal Bridge/RConn2
  Three-Phase Transformer (Two Windings)/RConn2 -- Three-Phase V-I Measurement5/LConn2
  Three-Phase V-I Measurement5/RConn3 -- Universal Bridge/LConn3
  Three-Phase V-I Measurement5/RConn1 -- Universal Bridge/LConn1
  Three-Phase Transformer (Two Windings)/RConn3 -- Three-Phase V-I Measurement5/LConn3
  Three-Phase V-I Measurement6/LConn1 -- Three-Phase Series RLC Branch/RConn1
  Three-Phase Series RLC Branch/RConn2 -- Three-Phase V-I Measurement6/LConn2
  Universal Bridge1/LConn1 -- Three-Phase V-I Measurement6/RConn1
  Three-Phase Series RLC Branch/RConn3 -- Three-Phase V-I Measurement6/LConn3
  Three-Phase V-I Measurement5/RConn2 -- Universal Bridge/LConn2

== system Wind_Turbine_test/Wind Farm/Wind Turbine 3 ==
  " base " : Gain  Gain=-P_mech/Wind_P_nom  SaturateOnIntegerOverflow=on  OutDataTypeStr=Inherit: Same as input  ParamDataTypeStr=Inherit: Same as input
  Asynchronous Machine pu Units : spsAsynchronousMachinepuUnitsLib/Asynchronous Machine pu Units  RotorType=Wound  PresetModel=No  MechanicalLoad=Torque Tm  ShowDetailedParameters=on  ReferenceFrame=Rotor  Units=pu  MeasurementBus=off  NominalParameters=[1.15e7 500 60]  VoltageRatio=1  Stator=[0.023 0.18]  Rotor=[0.016 0.16]  Cage1=[0.01909 0.0397]  Cage2=[0.01909 0.0397]  Lm=2.9  Mechanical=[0.685,0.01,3]  PolePairs=2  InitialConditions="[ -0.2,0   0,0,0   0,0,0 ]"  SimulateSaturation=off  Saturation="[0.212,0.4201,0.8125,1.0979,1.4799,2.2457,3.2586,4.5763,6.4763 ;   0.5,0.7,0.9,1,1.1,1.2 ,1.3,1.4,1.5]"  LoadFlowParameters=0  TsPowergui=0  TsBlock=-1  IterativeModel=Trapezoidal non iterative  IterativeDiscreteModel=Trapezoidal non iterative  Pmec=1.08e6
      settings: LibrarySourceBlock=|
      | sps_lib/Electrical Machines/Asynchronous Machine
      | pu Units
  Bus Selector : BusSelector  OutputSignals=Stator measurements.Stator current is_a (pu),Stator measurements.Stator current is_b (pu),Stator measurements.Stator current is_c (pu),Rotor measurements.Rotor current ir_a (pu),Rotor measurements.Rotor current ir_b (pu),Rotor measurements.Rotor current ir_c (pu),Mechanical.Electromagnetic torque Te (pu),Mechanical.Rotor speed (wm),Mechanical.Rotor angle thetam (rad)
  Mux : Mux  Inputs=3
  Mux1 : Mux  Inputs=3
  Series RLC Branch4 : spsSeriesRLCBranchLib/Series RLC Branch  LConnTagsString=__new0  RConnTagsString=__new0  BranchType=C  Resistance=1  Inductance=1e-3  SetiL0=off  InitialCurrent=0  Capacitance=0.06  Setx0=on  InitialVoltage=1175  Measurements=None
  Three-Phase Series RLC Branch : spsThreePhaseSeriesRLCBranchLib/Three-Phase Series RLC Branch  LConnTagsString=A|B|C  RConnTagsString=A|B|C  BranchType=RL  Resistance=(Wind_V_nom^2/Wind_P_nom)*R_pu  Inductance=(Wind_V_nom^2/Wind_P_nom/(2*pi*Wind_Freq_nom))*L_pu  Capacitance=1e-6  Measurements=None
  Three-Phase Transformer (Two Windings) : spsThreePhaseTransformerTwoWindingsLib/Three-Phase Transformer (Two Windings)  Winding1Connection=Y  Winding2Connection=Y  CoreType=Three single-phase transformers  SetSaturation=off  Hysteresis=off  DataFile='hysteresis'  SetInitialFlux=off  Measurements=None  UNITS=pu  NominalPower=[1.15e7, 60 ]  Winding1="[ 500, 0,0  ]"  Winding2=[ 1950 , 0 , 0 ]  Rm=500  Lm=inf  L0=0.5  Saturation=[ 0,0 ; 0.0024,1.2 ; 1.0,1.52 ]  InitialFluxes=[ 0.8 , -0.8 , 0.7 ]  BreakLoop=off  DiscreteSolver=Trapezoidal iterative  DataType=off  TransfoNumber=1
  Three-Phase V-I Measurement5 : spsThreePhaseVIMeasurementLib/Three-Phase V-I Measurement  VoltageMeasurement=phase-to-ground  SetLabelV=on  LabelV=Rotor_Vabc_WT3  Vpu=on  VpuLL=off  CurrentMeasurement=no  SetLabelI=on  LabelI=Iabc_WT1  Ipu=on  Pbase=2*1.8/0.9  Vbase=Wind_Rotor_V_nom  OutputType=Complex  PhasorSimulation=off  PSBequivalent=0
  Three-Phase V-I Measurement6 : spsThreePhaseVIMeasurementLib/Three-Phase V-I Measurement  VoltageMeasurement=phase-to-ground  SetLabelV=on  LabelV=Grid_conv_Vabc_WT3  Vpu=on  VpuLL=off  CurrentMeasurement=yes  SetLabelI=on  LabelI=Grid_conv_Iabc_WT3  Ipu=on  Pbase=1.15e7  Vbase=Wind_V_nom  OutputType=Complex  PhasorSimulation=off  PSBequivalent=0
  Universal Bridge : spsUniversalBridgeLib/Universal Bridge  Arms=3  SnubberResistance=1e3  SnubberCapacitance=inf  Device=IGBT / Diodes  Ron=1e-4/WT_IGBTRon  Lon=0  ForwardVoltages="[  0  0  ]"  ForwardVoltage=0  GTOparameters=[ 10e-6 , 20e-6 ]  IGBTparameters=[ 1e-6 , 2e-6 ]  Measurements=None  Measurements_2=None  converterType=Rectifier
  Universal Bridge1 : spsUniversalBridgeLib/Universal Bridge  Arms=3  SnubberResistance=1e3  SnubberCapacitance=inf  Device=IGBT / Diodes  Ron=1e-4/WT_IGBTRon  Lon=0  ForwardVoltages="[  0  0  ]"  ForwardVoltage=0  GTOparameters=[ 10e-6 , 20e-6 ]  IGBTparameters=[ 1e-6 , 2e-6 ]  Measurements=None  Measurements_2=None  converterType=Rectifier
  Wind Turbine & Generator 1 : Subsystem
  A : PMIOPort  Side=Left
  B : PMIOPort  Port=2  Side=Left
  C : PMIOPort  Port=3  Side=Left
  tag scope: Rotor_Angle_WT3=global, Rotor_Iabc_WT3=global, Rotor_Tem_WT3=global, Rotor_wm_WT3=global, Stator_Iabc_WT3=global, Tshaft_WT3=global, m_WT3=global
  wires:
  [Tshaft_WT3] -> Asynchronous Machine pu Units/1
  Wind Turbine & Generator 1/1(T_shaft (pu)) -> " base "/1
  " base "/1 -> [Tshaft_WT3]
  Asynchronous Machine pu Units/1 -> [m_WT3]
  [Grid_conv_pulses_WT3] -> Universal Bridge1/1
  [Rotor_conv_pulses_WT3] -> Universal Bridge/1
  [Rotor_wm_WT3] -> Wind Turbine & Generator 1/1(Generator speed (pu))
  [m_WT3] -> Bus Selector/1
  Bus Selector/1 -> Mux1/1  "<Stator current is_a (pu)>"
  Bus Selector/2 -> Mux1/2  "<Stator current is_b (pu)>"
  Bus Selector/3 -> Mux1/3  "<Stator current is_c (pu)>"
  Bus Selector/4 -> Mux/1  "<Rotor current ir_a (pu)>"
  Bus Selector/5 -> Mux/2  "<Rotor current ir_b (pu)>"
  Bus Selector/6 -> Mux/3  "<Rotor current ir_c (pu)>"
  Bus Selector/7 -> [Rotor_Tem_WT3]  "<Electromagnetic torque Te (pu)>"
  Bus Selector/8 -> [Rotor_wm_WT3]  "<Rotor speed (wm)>"
  Bus Selector/9 -> [Rotor_Angle_WT3]  "<Rotor angle thetam (rad)>"
  Mux/1 -> [Rotor_Iabc_WT3]
  Mux1/1 -> [Stator_Iabc_WT3]
  connections:
  Asynchronous Machine pu Units/LConn3 -- C/RConn1 -- Three-Phase Series RLC Branch/LConn3
  Three-Phase Series RLC Branch/LConn1 -- A/RConn1 -- Asynchronous Machine pu Units/LConn1
  Three-Phase Transformer (Two Windings)/LConn1 -- Asynchronous Machine pu Units/RConn1
  Three-Phase Transformer (Two Windings)/RConn1 -- Three-Phase V-I Measurement5/LConn1
  Three-Phase Series RLC Branch/LConn2 -- B/RConn1 -- Asynchronous Machine pu Units/LConn2
  Universal Bridge1/LConn3 -- Three-Phase V-I Measurement6/RConn3
  Three-Phase Transformer (Two Windings)/LConn3 -- Asynchronous Machine pu Units/RConn3
  Three-Phase Transformer (Two Windings)/LConn2 -- Asynchronous Machine pu Units/RConn2
  Universal Bridge1/LConn2 -- Three-Phase V-I Measurement6/RConn2
  Universal Bridge/RConn1 -- Series RLC Branch4/LConn1 -- Universal Bridge1/RConn1
  Universal Bridge1/RConn2 -- Series RLC Branch4/RConn1 -- Universal Bridge/RConn2
  Three-Phase Transformer (Two Windings)/RConn2 -- Three-Phase V-I Measurement5/LConn2
  Three-Phase V-I Measurement5/RConn3 -- Universal Bridge/LConn3
  Three-Phase V-I Measurement5/RConn1 -- Universal Bridge/LConn1
  Three-Phase Transformer (Two Windings)/RConn3 -- Three-Phase V-I Measurement5/LConn3
  Three-Phase V-I Measurement6/LConn1 -- Three-Phase Series RLC Branch/RConn1
  Three-Phase Series RLC Branch/RConn2 -- Three-Phase V-I Measurement6/LConn2
  Universal Bridge1/LConn1 -- Three-Phase V-I Measurement6/RConn1
  Three-Phase Series RLC Branch/RConn3 -- Three-Phase V-I Measurement6/LConn3
  Three-Phase V-I Measurement5/RConn2 -- Universal Bridge/LConn2

== system Wind_Turbine_test/Wind Farm/Wind Turbine 4 ==
  " base " : Gain  Gain=-P_mech/Wind_P_nom  SaturateOnIntegerOverflow=on  OutDataTypeStr=Inherit: Same as input  ParamDataTypeStr=Inherit: Same as input
  Asynchronous Machine pu Units : spsAsynchronousMachinepuUnitsLib/Asynchronous Machine pu Units  RotorType=Wound  PresetModel=No  MechanicalLoad=Torque Tm  ShowDetailedParameters=on  ReferenceFrame=Rotor  Units=pu  MeasurementBus=off  NominalParameters=[1.15e7 500 60]  VoltageRatio=1  Stator=[0.023 0.18]  Rotor=[0.016 0.16]  Cage1=[0.01909 0.0397]  Cage2=[0.01909 0.0397]  Lm=2.9  Mechanical=[0.685,0.01,3]  PolePairs=2  InitialConditions="[ -0.2,0   0,0,0   0,0,0 ]"  SimulateSaturation=off  Saturation="[0.212,0.4201,0.8125,1.0979,1.4799,2.2457,3.2586,4.5763,6.4763 ;   0.5,0.7,0.9,1,1.1,1.2 ,1.3,1.4,1.5]"  LoadFlowParameters=0  TsPowergui=0  TsBlock=-1  IterativeModel=Trapezoidal non iterative  IterativeDiscreteModel=Trapezoidal non iterative  Pmec=1.08e6
      settings: LibrarySourceBlock=|
      | sps_lib/Electrical Machines/Asynchronous Machine
      | pu Units
  Bus Selector : BusSelector  OutputSignals=Stator measurements.Stator current is_a (pu),Stator measurements.Stator current is_b (pu),Stator measurements.Stator current is_c (pu),Rotor measurements.Rotor current ir_a (pu),Rotor measurements.Rotor current ir_b (pu),Rotor measurements.Rotor current ir_c (pu),Mechanical.Electromagnetic torque Te (pu),Mechanical.Rotor speed (wm),Mechanical.Rotor angle thetam (rad)
  Mux : Mux  Inputs=3
  Mux1 : Mux  Inputs=3
  Series RLC Branch4 : spsSeriesRLCBranchLib/Series RLC Branch  LConnTagsString=__new0  RConnTagsString=__new0  BranchType=C  Resistance=1  Inductance=1e-3  SetiL0=off  InitialCurrent=0  Capacitance=0.06  Setx0=on  InitialVoltage=1175  Measurements=None
  Three-Phase Series RLC Branch : spsThreePhaseSeriesRLCBranchLib/Three-Phase Series RLC Branch  LConnTagsString=A|B|C  RConnTagsString=A|B|C  BranchType=RL  Resistance=(Wind_V_nom^2/Wind_P_nom)*R_pu  Inductance=(Wind_V_nom^2/Wind_P_nom/(2*pi*Wind_Freq_nom))*L_pu  Capacitance=1e-6  Measurements=None
  Three-Phase Transformer (Two Windings) : spsThreePhaseTransformerTwoWindingsLib/Three-Phase Transformer (Two Windings)  Winding1Connection=Y  Winding2Connection=Y  CoreType=Three single-phase transformers  SetSaturation=off  Hysteresis=off  DataFile='hysteresis'  SetInitialFlux=off  Measurements=None  UNITS=pu  NominalPower=[1.15e7, 60 ]  Winding1="[ 500, 0,0  ]"  Winding2=[ 1950 , 0 , 0 ]  Rm=500  Lm=inf  L0=0.5  Saturation=[ 0,0 ; 0.0024,1.2 ; 1.0,1.52 ]  InitialFluxes=[ 0.8 , -0.8 , 0.7 ]  BreakLoop=off  DiscreteSolver=Trapezoidal iterative  DataType=off  TransfoNumber=1
  Three-Phase V-I Measurement5 : spsThreePhaseVIMeasurementLib/Three-Phase V-I Measurement  VoltageMeasurement=phase-to-ground  SetLabelV=on  LabelV=Rotor_Vabc_WT4  Vpu=on  VpuLL=off  CurrentMeasurement=no  SetLabelI=on  LabelI=Iabc_WT1  Ipu=on  Pbase=2*1.8/0.9  Vbase=Wind_Rotor_V_nom  OutputType=Complex  PhasorSimulation=off  PSBequivalent=0
  Three-Phase V-I Measurement6 : spsThreePhaseVIMeasurementLib/Three-Phase V-I Measurement  VoltageMeasurement=phase-to-ground  SetLabelV=on  LabelV=Grid_conv_Vabc_WT4  Vpu=on  VpuLL=off  CurrentMeasurement=yes  SetLabelI=on  LabelI=Grid_conv_Iabc_WT4  Ipu=on  Pbase=1.15e7  Vbase=Wind_V_nom  OutputType=Complex  PhasorSimulation=off  PSBequivalent=0
  Universal Bridge : spsUniversalBridgeLib/Universal Bridge  Arms=3  SnubberResistance=1e3  SnubberCapacitance=inf  Device=IGBT / Diodes  Ron=1e-4/WT_IGBTRon  Lon=0  ForwardVoltages="[  0  0  ]"  ForwardVoltage=0  GTOparameters=[ 10e-6 , 20e-6 ]  IGBTparameters=[ 1e-6 , 2e-6 ]  Measurements=None  Measurements_2=None  converterType=Rectifier
  Universal Bridge1 : spsUniversalBridgeLib/Universal Bridge  Arms=3  SnubberResistance=1e3  SnubberCapacitance=inf  Device=IGBT / Diodes  Ron=1e-4/WT_IGBTRon  Lon=0  ForwardVoltages="[  0  0  ]"  ForwardVoltage=0  GTOparameters=[ 10e-6 , 20e-6 ]  IGBTparameters=[ 1e-6 , 2e-6 ]  Measurements=None  Measurements_2=None  converterType=Rectifier
  Wind Turbine & Generator 1 : Subsystem
  A : PMIOPort  Side=Left
  B : PMIOPort  Port=2  Side=Left
  C : PMIOPort  Port=3  Side=Left
  tag scope: Rotor_Angle_WT4=global, Rotor_Iabc_WT4=global, Rotor_Tem_WT4=global, Rotor_wm_WT4=global, Stator_Iabc_WT4=global, Tshaft_WT4=global, m_WT4=global
  wires:
  [Tshaft_WT4] -> Asynchronous Machine pu Units/1
  Wind Turbine & Generator 1/1(T_shaft (pu)) -> " base "/1
  " base "/1 -> [Tshaft_WT4]
  Asynchronous Machine pu Units/1 -> [m_WT4]
  [Grid_conv_pulses_WT4] -> Universal Bridge1/1
  [Rotor_conv_pulses_WT4] -> Universal Bridge/1
  [Rotor_wm_WT4] -> Wind Turbine & Generator 1/1(Generator speed (pu))
  [m_WT4] -> Bus Selector/1
  Bus Selector/1 -> Mux1/1  "<Stator current is_a (pu)>"
  Bus Selector/2 -> Mux1/2  "<Stator current is_b (pu)>"
  Bus Selector/3 -> Mux1/3  "<Stator current is_c (pu)>"
  Bus Selector/4 -> Mux/1  "<Rotor current ir_a (pu)>"
  Bus Selector/5 -> Mux/2  "<Rotor current ir_b (pu)>"
  Bus Selector/6 -> Mux/3  "<Rotor current ir_c (pu)>"
  Bus Selector/7 -> [Rotor_Tem_WT4]  "<Electromagnetic torque Te (pu)>"
  Bus Selector/8 -> [Rotor_wm_WT4]  "<Rotor speed (wm)>"
  Bus Selector/9 -> [Rotor_Angle_WT4]  "<Rotor angle thetam (rad)>"
  Mux/1 -> [Rotor_Iabc_WT4]
  Mux1/1 -> [Stator_Iabc_WT4]
  connections:
  Asynchronous Machine pu Units/LConn3 -- C/RConn1 -- Three-Phase Series RLC Branch/LConn3
  Three-Phase Series RLC Branch/LConn1 -- A/RConn1 -- Asynchronous Machine pu Units/LConn1
  Three-Phase Transformer (Two Windings)/LConn1 -- Asynchronous Machine pu Units/RConn1
  Three-Phase Transformer (Two Windings)/RConn1 -- Three-Phase V-I Measurement5/LConn1
  Three-Phase Series RLC Branch/LConn2 -- B/RConn1 -- Asynchronous Machine pu Units/LConn2
  Universal Bridge1/LConn3 -- Three-Phase V-I Measurement6/RConn3
  Three-Phase Transformer (Two Windings)/LConn3 -- Asynchronous Machine pu Units/RConn3
  Three-Phase Transformer (Two Windings)/LConn2 -- Asynchronous Machine pu Units/RConn2
  Universal Bridge1/LConn2 -- Three-Phase V-I Measurement6/RConn2
  Universal Bridge/RConn1 -- Series RLC Branch4/LConn1 -- Universal Bridge1/RConn1
  Universal Bridge1/RConn2 -- Series RLC Branch4/RConn1 -- Universal Bridge/RConn2
  Three-Phase Transformer (Two Windings)/RConn2 -- Three-Phase V-I Measurement5/LConn2
  Three-Phase V-I Measurement5/RConn3 -- Universal Bridge/LConn3
  Three-Phase V-I Measurement5/RConn1 -- Universal Bridge/LConn1
  Three-Phase Transformer (Two Windings)/RConn3 -- Three-Phase V-I Measurement5/LConn3
  Three-Phase V-I Measurement6/LConn1 -- Three-Phase Series RLC Branch/RConn1
  Three-Phase Series RLC Branch/RConn2 -- Three-Phase V-I Measurement6/LConn2
  Universal Bridge1/LConn1 -- Three-Phase V-I Measurement6/RConn1
  Three-Phase Series RLC Branch/RConn3 -- Three-Phase V-I Measurement6/LConn3
  Three-Phase V-I Measurement5/RConn2 -- Universal Bridge/LConn2
